simulink model "Cruise_Control_PI_Control"  (R2017b)
settings: Solver=VariableStepAuto  StartTime=0.0  StopTime=50  RelTol=1e-3
values from neighbouring files (symbols this model uses):
  a = 200    [CruiseControl_param.m]    (also in Example_VehicleSteering_PP.m = 2)
  b = 10000    [CruiseControl_param.m]    (also in Example_VehicleSteering_PP.m = 4)
  ki = 0.07    [CruiseControl_param.m]
  kp = 0.1    [CruiseControl_param.m]
  m = 1000    [CruiseControl_param.m]
settings Model: Creator=rizwanahmed  LastModifiedBy=rizwanahmed

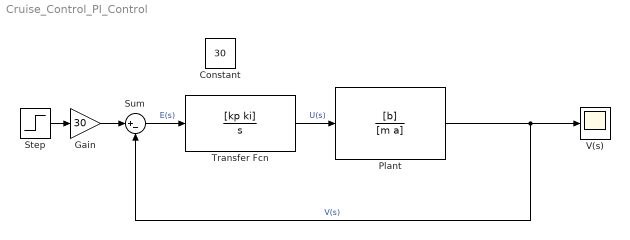
== system Cruise_Control_PI_Control ==
  " Plant" : TransferFcn  Numerator=[b]  Denominator=[m a]
  Constant : Constant  Value=30
  Gain : Gain  Gain=30
  Step : Step  Time=20  SampleTime=0
  Sum : Sum  Inputs=|+-
  Transfer Fcn : TransferFcn  Numerator=[kp ki]  Denominator=[1 0]
  V(s) : Scope
  wires:
  " Plant"/1 -> Sum/2, V(s)/1  "V(s)"
  Transfer Fcn/1 -> " Plant"/1  "U(s)"
  Sum/1 -> Transfer Fcn/1  "E(s)"
  Step/1 -> Gain/1
  Gain/1 -> Sum/1
